simulink model "Planta_1"  (Simulink 7.9)
settings: Solver=ode45  StartTime=0.0  StopTime=10.0  RelTol=1e-3
settings Model: Creator=Carlos  LastModifiedBy=Carlos

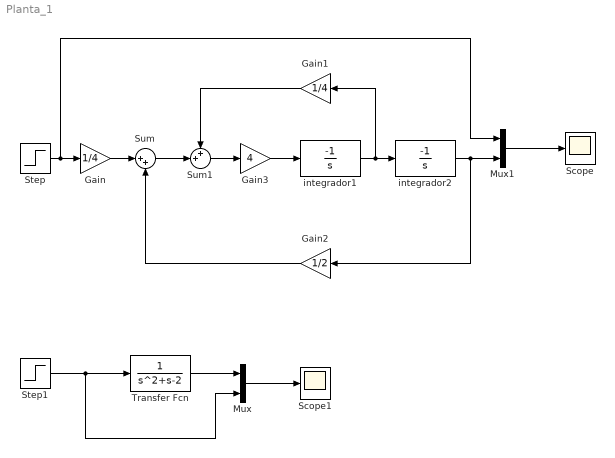
== system Planta_1 ==
  Gain : Gain  Gain=1/4
  Gain1 : Gain  Gain=1/4
  Gain2 : Gain  Gain=1/2
  Gain3 : Gain  Gain=4
  Mux : Mux  Inputs=2
  Mux1 : Mux  Inputs=2
  Scope : Scope
      settings: YMin=-0.5  YMax=11
  Scope1 : Scope
      settings: TimeRange=10  YMin=-0.5  YMax=11
  Step : Step  SampleTime=0
  Step1 : Step  SampleTime=0
  Sum : Sum  Inputs=|++
  Sum1 : Sum  Inputs=++|
  Transfer Fcn : TransferFcn  Denominator=[1 1 -2]
  integrador1 : TransferFcn  Numerator=[-1]  Denominator=[1 0]
  integrador2 : TransferFcn  Numerator=[-1]  Denominator=[1 0]
  wires:
  Step/1 -> Gain/1, Mux1/1
  Gain/1 -> Sum/1
  Gain2/1 -> Sum/2
  Gain1/1 -> Sum1/1
  Sum1/1 -> Gain3/1
  Sum/1 -> Sum1/2
  Step1/1 -> Transfer Fcn/1, Mux/2
  Gain3/1 -> integrador1/1
  integrador1/1 -> integrador2/1, Gain1/1
  integrador2/1 -> Mux1/2, Gain2/1
  Mux1/1 -> Scope/1
  Transfer Fcn/1 -> Mux/1
  Mux/1 -> Scope1/1
